simulink model "smib_r2008b_start_simple"  (Simulink 7.2)
settings: Solver=ode3  StartTime=0.0  StopTime=15  FixedStep=1e-4  MaxStep=1e-4  RelTol=1e-4
values from neighbouring files (symbols this model uses):
  D = 0.01    [MODEL_WORKSPACE.mat]    (also in MODEL_WORKSPACE_53.mat; WS.mat)
  J = 20    [MODEL_WORKSPACE.mat]    (also in MODEL_WORKSPACE_53.mat; WS.mat)
  Rf = 0.00246    [MODEL_WORKSPACE.mat]    (also in MODEL_WORKSPACE_53.mat = 0.0025; WS.mat = 0.0025)
  Tdo = 3    [MODEL_WORKSPACE.mat]    (also in MODEL_WORKSPACE_53.mat; WS.mat)
  X = 0.4    [MODEL_WORKSPACE.mat]    (also in MODEL_WORKSPACE_53.mat; WS.mat)
  Xd = 1    [MODEL_WORKSPACE.mat]    (also in MODEL_WORKSPACE_53.mat; WS.mat)
  Xdp = 0.25    [MODEL_WORKSPACE.mat]    (also in MODEL_WORKSPACE_53.mat; WS.mat)
  Xf = 0.8    [MODEL_WORKSPACE.mat]    (also in MODEL_WORKSPACE_53.mat; WS.mat)
libraries: simulink x1
settings Model: Creator=Admin  LastModifiedBy=Admin  ExtModeTrigMode=oneshot  ExtModeArmWhenConnect=off
settings DataIOCC: LimitDataPoints=off
settings OptimizationCC: BlockReduction=off  BooleanDataType=off
settings DebuggingCC: SaveWithParameterizedLinksMsg=none  SignalResolutionControl=TryResolveAllWithWarning  SolverPrmCheckMsg=none  MultiTaskDSMMsg=warning  MultiTaskCondExecSysMsg=none  StrictBusMsg=None
settings HardwareCC: TargetUnknown=on
settings RTWCC: IncludeERTFirstTime=on
settings GRTTargetCC: ModelReferenceCompliant=off  CompOptLevelCompliant=off  MatFileLogging=off

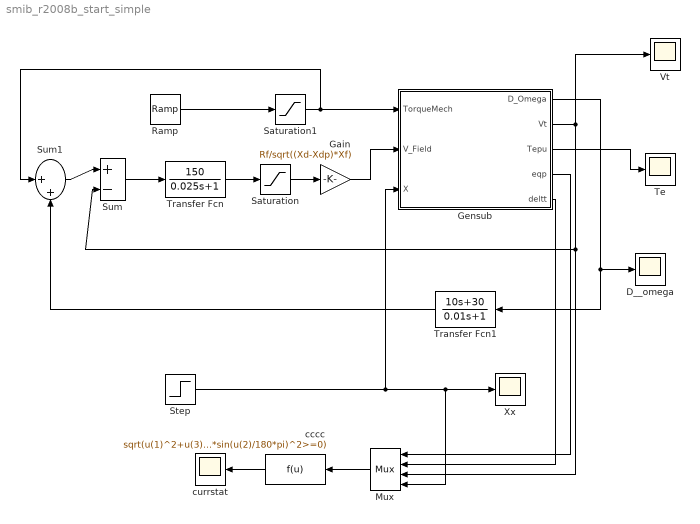
== system smib_r2008b_start_simple ==
  D__omega : Scope
      settings: YMin=0  YMax=0.003  MaxDataPoints=500000
  Gain : Gain  Gain=Rf/sqrt((Xd-Xdp)*Xf)  SaturateOnIntegerOverflow=on  OutDataTypeStr=Inherit: Same as input  ParamDataTypeStr=Inherit: Same as input
  Gensub : Subsystem
  Mux : Mux  Orientation=left
  Ramp : simulink/Sources/Ramp  SystemSampleTime=-1  slope=0.3  start=0  X0=0
  Saturation : Saturate  UpperLimit=1.9  LowerLimit=0
  Saturation1 : Saturate  UpperLimit=1  LowerLimit=0
  Step : Step  Time=0.9  Before=10000000*X  After=X  SampleTime=0
  Sum : Sum  Inputs=|+-  SaturateOnIntegerOverflow=on  InputSameDT=on  OutDataTypeStr=Inherit: Same as first input
  Sum1 : Sum  Inputs=|++  SaturateOnIntegerOverflow=on  InputSameDT=on  OutDataTypeStr=Inherit: Same as first input
  Te : Scope
      settings: YMin=-0.5  YMax=1.5  MaxDataPoints=500000
  Transfer Fcn : TransferFcn  Numerator=[150]  Denominator=[0.025 1]
  Transfer Fcn1 : TransferFcn  Orientation=left  Numerator=[10 30]  Denominator=[0.01 1]
  Vt : Scope
      settings: YMin=0  YMax=1.25  MaxDataPoints=500000
  Xx : Scope
      settings: YMin=0  YMax=4000  MaxDataPoints=500000
  cccc : Fcn  Orientation=left  Expr=sqrt(u(1)^2+u(3)^2-2*u(1)*u(3)*cos(u(2)/180*pi))/Xdp*(Vbus^2/u(4)^2-u(1)^2/Xdp^2*sin(u(2)/180*pi)^2>=0)
  currstat : Scope
      settings: YMin=0  YMax=2.5  MaxDataPoints=500000
  wires:
  Gain/1 -> Gensub/2(V_Field)
  Saturation/1 -> Gain/1
  Transfer Fcn/1 -> Saturation/1
  Sum/1 -> Transfer Fcn/1
  Sum1/1 -> Sum/1
  Gensub/2(Vt) -> Vt/1, Sum/2, Mux/3
  Gensub/3(Tepu) -> Te/1
  Saturation1/1 -> Gensub/1(TorqueMech), Sum1/1
  Gensub/1(D_Omega) -> D__omega/1, Transfer Fcn1/1
  Step/1 -> Gensub/3(X), Xx/1, Mux/4
  Transfer Fcn1/1 -> Sum1/2
  Gensub/4(eqp) -> Mux/1
  Gensub/5(deltt) -> Mux/2
  Mux/1 -> cccc/1
  cccc/1 -> currstat/1
  Ramp/1 -> Saturation1/1

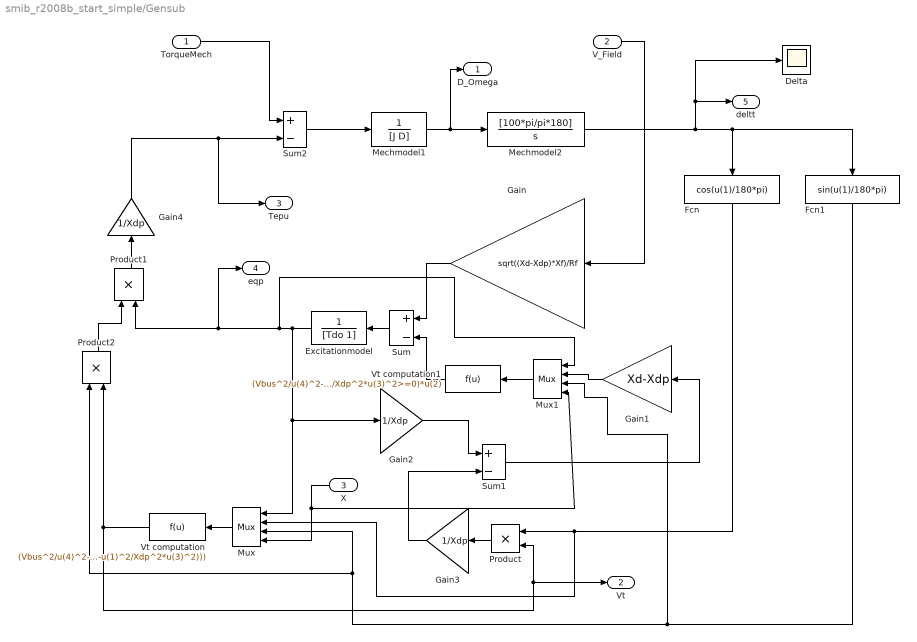
== system smib_r2008b_start_simple/Gensub ==
  TorqueMech : Inport
  V_Field : Inport  Port=2
  X : Inport  Orientation=left  Port=3
  Delta : Scope
      settings: YMin=-10  YMax=60  MaxDataPoints=500000
  Excitationmodel : TransferFcn  Orientation=left  Denominator=[Tdo 1]
  Fcn : Fcn  Orientation=down  Expr=cos(u(1)/180*pi)
  Fcn1 : Fcn  Orientation=down  Expr=sin(u(1)/180*pi)
  Gain : Gain  Orientation=left  Gain=sqrt((Xd-Xdp)*Xf)/Rf  SaturateOnIntegerOverflow=on  OutDataTypeStr=Inherit: Same as input  ParamDataTypeStr=Inherit: Same as input
  Gain1 : Gain  Orientation=left  Gain=Xd-Xdp  SaturateOnIntegerOverflow=on  OutDataTypeStr=Inherit: Same as input  ParamDataTypeStr=Inherit: Same as input
  Gain2 : Gain  Gain=1/Xdp  SaturateOnIntegerOverflow=on  OutDataTypeStr=Inherit: Same as input  ParamDataTypeStr=Inherit: Same as input
  Gain3 : Gain  Orientation=left  Gain=1/Xdp  SaturateOnIntegerOverflow=on  OutDataTypeStr=Inherit: Same as input  ParamDataTypeStr=Inherit: Same as input
  Gain4 : Gain  Orientation=up  Gain=1/Xdp  SaturateOnIntegerOverflow=on  OutDataTypeStr=Inherit: Same as input  ParamDataTypeStr=Inherit: Same as input
  Mechmodel1 : TransferFcn  Denominator=[J D]
  Mechmodel2 : TransferFcn  Numerator=[100*pi/pi*180]  Denominator=[1 0]
  Mux : Mux  Orientation=left
  Mux1 : Mux  Orientation=left
  Product : Product  Orientation=left  SaturateOnIntegerOverflow=on  RndMeth=Zero  InputSameDT=on  OutDataTypeStr=Inherit: Same as first input
  Product1 : Product  Orientation=up  SaturateOnIntegerOverflow=on  RndMeth=Zero  InputSameDT=on  OutDataTypeStr=Inherit: Same as first input
  Product2 : Product  Orientation=up  SaturateOnIntegerOverflow=on  RndMeth=Zero  InputSameDT=on  OutDataTypeStr=Inherit: Same as first input
  Sum : Sum  Orientation=left  Inputs=|+-  SaturateOnIntegerOverflow=on  InputSameDT=on  OutDataTypeStr=Inherit: Same as first input
  Sum1 : Sum  Inputs=|+-  SaturateOnIntegerOverflow=on  InputSameDT=on  OutDataTypeStr=Inherit: Same as first input
  Sum2 : Sum  Inputs=|+-  SaturateOnIntegerOverflow=on  InputSameDT=on  OutDataTypeStr=Inherit: Same as first input
  Vt computation : Fcn  Orientation=left  Expr=(Vbus^2/u(4)^2-u(1)^2/Xdp^2*u(3)^2>=0)*1/(1/u(4)+1/Xdp)*(u(1)/Xdp*u(2)+sqrt(abs(Vbus^2/u(4)^2-u(1)^2/Xdp^2*u(3)^2)))
  Vt computation1 : Fcn  Orientation=left  Expr=(Vbus^2/u(4)^2-u(1)^2/Xdp^2*u(3)^2>=0)*u(2)
  D_Omega : Outport
  Vt : Outport  Port=2
  Tepu : Outport  Port=3
  eqp : Outport  Port=4
  deltt : Outport  Port=5
  wires:
  Mechmodel1/1 -> Mechmodel2/1, D_Omega/1
  V_Field/1 -> Gain/1
  Gain/1 -> Sum/1
  Sum1/1 -> Gain1/1
  Gain2/1 -> Sum1/1
  Gain3/1 -> Sum1/2
  Product/1 -> Gain3/1
  Sum/1 -> Excitationmodel/1
  Excitationmodel/1 -> Gain2/1, Mux/1, Product1/2, eqp/1, Mux1/1
  Product2/1 -> Product1/1
  Fcn/1 -> Product/1, Mux/2
  Fcn1/1 -> Mux/3, Product2/1, Mux1/3
  Vt computation/1 -> Product2/2, Product/2, Vt/1
  Product1/1 -> Gain4/1
  Sum2/1 -> Mechmodel1/1
  TorqueMech/1 -> Sum2/1
  Gain4/1 -> Sum2/2, Tepu/1
  X/1 -> Mux/4, Mux1/4
  Mechmodel2/1 -> Fcn/1, Fcn1/1, Delta/1, deltt/1
  Mux/1 -> Vt computation/1
  Vt computation1/1 -> Sum/2
  Mux1/1 -> Vt computation1/1
  Gain1/1 -> Mux1/2
